simulink model "rob_zadanie2_sim1"  (R2023b)
settings: Solver=VariableStepAuto  StartTime=0.0  StopTime=50  RelTol=1e-3
undefined symbols (not defined in the file or in its folder): B1, B2, g, l1, l2, m1, m2
settings Model: Creator=Filip  LastModifiedBy=Filip
settings DebuggingCC: AlgebraicLoopMsg=none

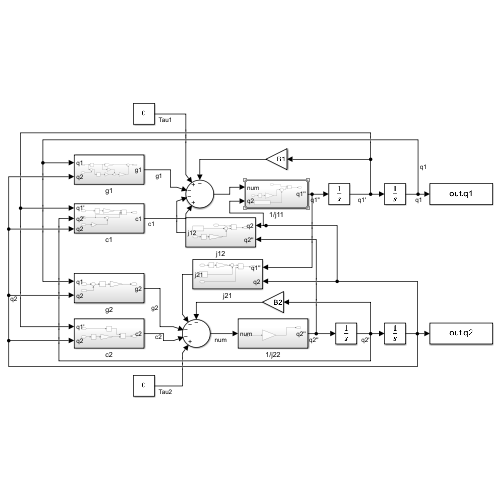
[thumbnail: Simulink's stored preview of the top-level diagram]
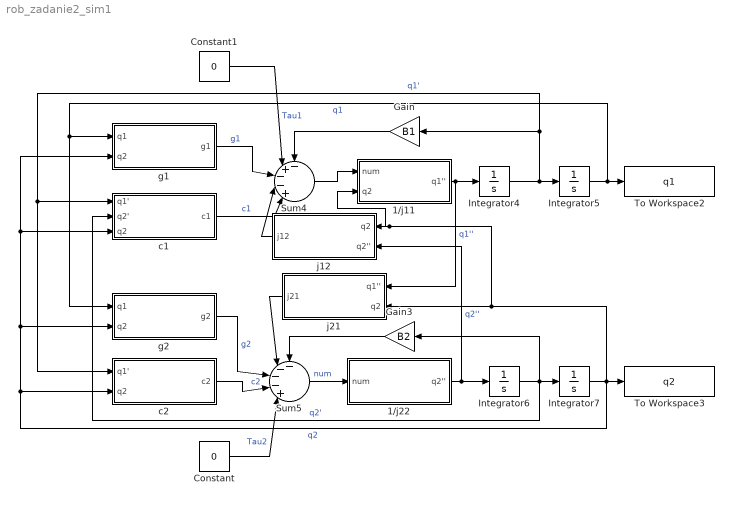
== system rob_zadanie2_sim1 ==
  1/j11 : Subsystem
  1/j22 : Subsystem
  Constant : Constant  Value=0
  Constant1 : Constant  Value=0
  Gain : Gain  Gain=B1
  Gain3 : Gain  Gain=B2
  Integrator{4..7} (4 alike) : Integrator
  Sum4 : Sum  Inputs=-+--+|
  Sum5 : Sum  Inputs=----+|
  To Workspace2 : ToWorkspace  VariableName=q1  SampleTime=-1
  To Workspace3 : ToWorkspace  VariableName=q2  SampleTime=-1
  c1 : Subsystem
  c2 : Subsystem
  g1 : Subsystem
  g2 : Subsystem
  j12 : Subsystem
  j21 : Subsystem
  wires:
  Constant/1 -> Sum5/5  "Tau2"
  Gain3/1 -> Sum5/1
  1/j11/1(q1'') -> j21/1(q1''), Integrator4/1  "q1''"
  Integrator7/1 -> To Workspace3/1, 1/j11/2(q2), j12/1(q2), j21/2(q2), g2/2(q2), g1/2(q2), c1/3(q2), c2/2(q2)  "q2"
  j21/1(j21) -> Sum5/2
  Constant1/1 -> Sum4/2  "Tau1"
  g2/1(g2) -> Sum5/3  "g2"
  Integrator5/1 -> To Workspace2/1, g2/1(q1), g1/1(q1)  "q1"
  Gain/1 -> Sum4/1
  Sum5/1 -> 1/j22/1(num)  "num"
  Integrator6/1 -> Gain3/1, c1/2(q2'), Integrator7/1  "q2'"
  g1/1(g1) -> Sum4/3  "g1"
  1/j22/1(q2'') -> j12/2(q2''), Integrator6/1  "q2''"
  c2/1(c2) -> Sum5/4  "c2"
  Sum4/1 -> 1/j11/1(num)
  Integrator4/1 -> Integrator5/1, c2/1(q1'), c1/1(q1'), Gain/1  "q1'"
  j12/1(j12) -> Sum4/4
  c1/1(c1) -> Sum4/5  "c1"

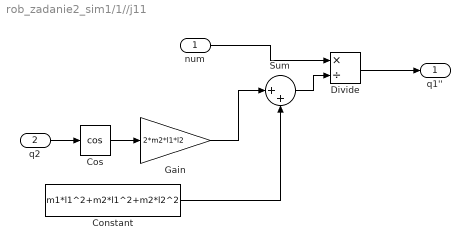
== system rob_zadanie2_sim1/1//j11 ==
  num : Inport
  q2 : Inport  Port=2
  Constant : Constant  Value=m1*l1^2+m2*l1^2+m2*l2^2
  Cos : Trigonometry  Operator=cos
  Divide : Product  Inputs=*/
  Gain : Gain  Gain=2*m2*l1*l2
  Sum : Sum  Inputs=|++
  q1'' : Outport
  wires:
  q2/1 -> Cos/1
  Cos/1 -> Gain/1
  Gain/1 -> Sum/1
  Constant/1 -> Sum/2
  num/1 -> Divide/1
  Sum/1 -> Divide/2
  Divide/1 -> q1''/1

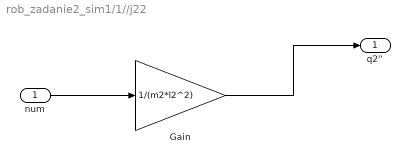
== system rob_zadanie2_sim1/1//j22 ==
  num : Inport
  Gain : Gain  Gain=1/(m2*l2^2)
  q2'' : Outport
  wires:
  num/1 -> Gain/1
  Gain/1 -> q2''/1

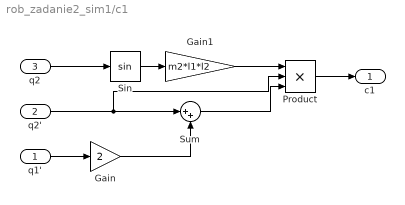
== system rob_zadanie2_sim1/c1 ==
  q1' : Inport
  q2' : Inport  Port=2
  q2 : Inport  Port=3
  Gain : Gain  Gain=2
  Gain1 : Gain  Gain=m2*l1*l2
  Product : Product  Inputs=3
  Sin : Trigonometry
  Sum : Sum  Inputs=|++
  c1 : Outport
  wires:
  q1'/1 -> Gain/1
  Gain/1 -> Sum/2
  q2'/1 -> Product/2, Sum/1
  q2/1 -> Sin/1
  Sin/1 -> Gain1/1
  Gain1/1 -> Product/1
  Product/1 -> c1/1
  Sum/1 -> Product/3

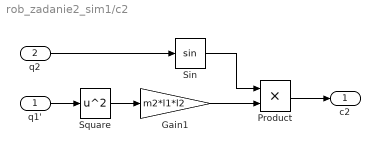
== system rob_zadanie2_sim1/c2 ==
  q1' : Inport
  q2 : Inport  Port=2
  Gain1 : Gain  Gain=m2*l1*l2
  Product : Product
  Sin : Trigonometry
  Square : Math  Operator=square
  c2 : Outport
  wires:
  q1'/1 -> Square/1
  Square/1 -> Gain1/1
  Gain1/1 -> Product/2
  q2/1 -> Sin/1
  Sin/1 -> Product/1
  Product/1 -> c2/1

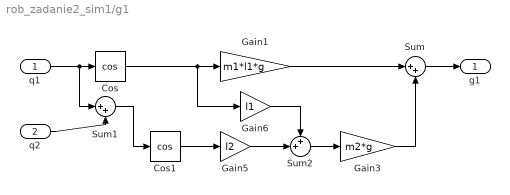
== system rob_zadanie2_sim1/g1 ==
  q1 : Inport
  q2 : Inport  Port=2
  Cos : Trigonometry  Operator=cos
  Cos1 : Trigonometry  Operator=cos
  Gain1 : Gain  Gain=m1*l1*g
  Gain3 : Gain  Gain=m2*g
  Gain5 : Gain  Gain=l2
  Gain6 : Gain  Gain=l1
  Sum : Sum  Inputs=|++
  Sum1 : Sum  Inputs=|++
  Sum2 : Sum  Inputs=++|
  g1 : Outport
  wires:
  q1/1 -> Sum1/1, Cos/1
  Cos/1 -> Gain1/1, Gain6/1
  q2/1 -> Sum1/2
  Sum1/1 -> Cos1/1
  Cos1/1 -> Gain5/1
  Gain5/1 -> Sum2/2
  Gain6/1 -> Sum2/1
  Sum2/1 -> Gain3/1
  Gain3/1 -> Sum/2
  Sum/1 -> g1/1
  Gain1/1 -> Sum/1

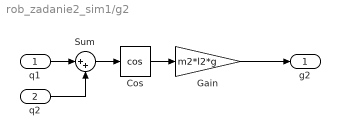
== system rob_zadanie2_sim1/g2 ==
  q1 : Inport
  q2 : Inport  Port=2
  Cos : Trigonometry  Operator=cos
  Gain : Gain  Gain=m2*l2*g
  Sum : Sum  Inputs=|++
  g2 : Outport
  wires:
  q1/1 -> Sum/1
  q2/1 -> Sum/2
  Sum/1 -> Cos/1
  Cos/1 -> Gain/1
  Gain/1 -> g2/1

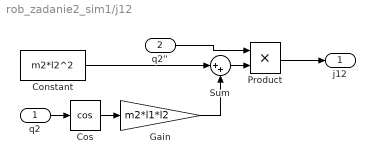
== system rob_zadanie2_sim1/j12 ==
  q2 : Inport
  q2'' : Inport  Port=2
  Constant : Constant  Value=m2*l2^2  SampleTime=-1
  Cos : Trigonometry  Operator=cos
  Gain : Gain  Gain=m2*l1*l2
  Product : Product
  Sum : Sum  Inputs=|++
  j12 : Outport
  wires:
  q2/1 -> Cos/1
  Cos/1 -> Gain/1
  Gain/1 -> Sum/2
  Constant/1 -> Sum/1
  Sum/1 -> Product/2
  q2''/1 -> Product/1
  Product/1 -> j12/1

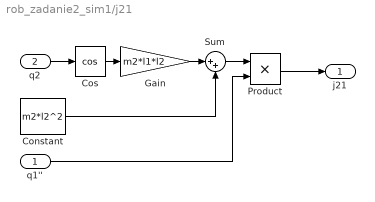
== system rob_zadanie2_sim1/j21 ==
  q1'' : Inport
  q2 : Inport  Port=2
  Constant : Constant  Value=m2*l2^2
  Cos : Trigonometry  Operator=cos
  Gain : Gain  Gain=m2*l1*l2
  Product : Product
  Sum : Sum  Inputs=|++
  j21 : Outport
  wires:
  q2/1 -> Cos/1
  Cos/1 -> Gain/1
  Gain/1 -> Sum/1
  Sum/1 -> Product/1
  q1''/1 -> Product/2
  Product/1 -> j21/1
  Constant/1 -> Sum/2
